simulink library "IAM_b0"  (Simulink 8.2)
settings: Solver=ode45  StartTime=0.0  StopTime=10.0  RelTol=1e-3
libraries: simulink x1, simulink_extras x1
settings Model: Creator=lena.frank  LastModifiedBy=drhf

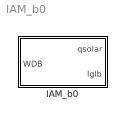
== system IAM_b0 ==
  IAM_b0 : Subsystem  mask(collector optics single glazing with extra white glass){fta=0.8, b0=0.12, Kd=0.92}
      mask prompts: fta "Fin Efficiency * Transmission * Absorption (FTA) [-]"; b0 "b0 : constant for the calculation of the incident angle modifier (direct radiation) [-]"; Kd "Kd : Incidence angle modifier diffuse radiation [-]"
      mask help:
      | USE IN THE "Collector_EN12975_FlatPlate" MODEL:
      | Transforms direct and diffuse radiation to an absorbed solar power per unit area. The direct radiation incidence angle modifier (Kdir) uses the b0-model for flat plate collectors (EN 12975).
      | FTA or F'(TauAlfa) is defined from the incidence angle modifiers Kdir and Kdfu:
      | FTA = eta0 / (Kdir(15°)*0.85 + Kdfu*0.15)
      mask Help: web(fullfile(path_carnot('help'),'IAM_b0.html'),'-helpbrowser')

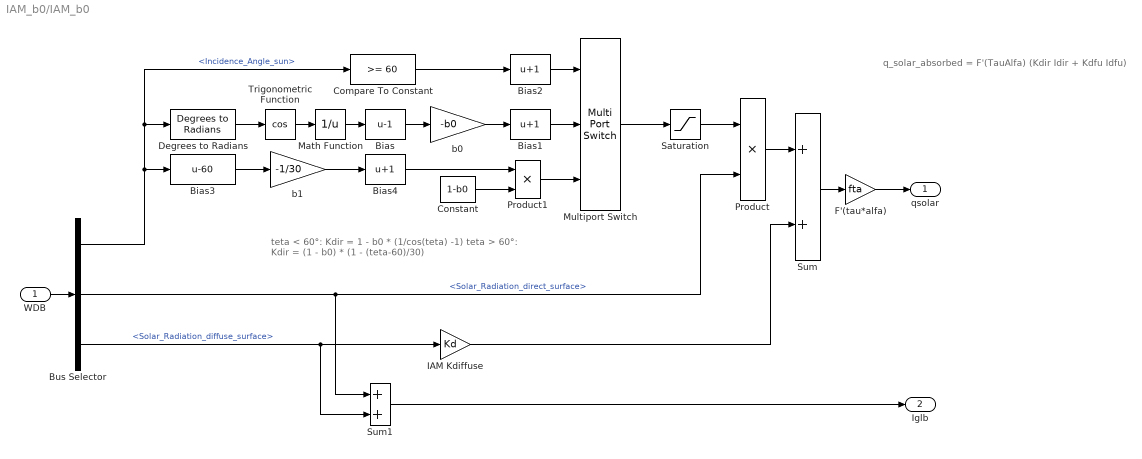
== system IAM_b0/IAM_b0 ==
  note: q_solar_absorbed = F'(TauAlfa) (Kdir Idir + Kdfu Idfu)
  note: teta < 60°: Kdir = 1 - b0 * (1/cos(teta) -1)
      | teta > 60°: Kdir = (1 - b0) * (1 - (teta-60)/30)
  WDB : Inport
  Bias : Bias  Bias=-1
  Bias1 : Bias  Bias=1
  Bias2 : Bias  Bias=1
  Bias3 : Bias  Bias=-60
  Bias4 : Bias  Bias=1
  Bus Selector : BusSelector  OutputSignals=Incidence_Angle_sun,Solar_Radiation_direct_surface,Solar_Radiation_diffuse_surface
  Compare To Constant : simulink/Logic and Bit Operations/Compare To Constant  relop=>=  const=60  OutDataTypeStr=uint8
  Constant : Constant  Value=1-b0
  Degrees to Radians : simulink_extras/Transformations/Degrees to Radians
  F'(tau*alfa) : Gain  Gain=fta  SaturateOnIntegerOverflow=on  OutDataTypeStr=Inherit: Same as input  ParamDataTypeStr=Inherit: Same as input
  IAM Kdiffuse : Gain  Gain=Kd  SaturateOnIntegerOverflow=on  OutDataTypeStr=Inherit: Same as input  ParamDataTypeStr=Inherit: Same as input
  Math Function : Math  Operator=reciprocal  SaturateOnIntegerOverflow=on
  Multiport Switch : MultiPortSwitch  Inputs=2
  Product : Product  RndMeth=Zero
  Product1 : Product  RndMeth=Zero
  Saturation : Saturate  UpperLimit=inf  LowerLimit=0
  Sum : Sum  SaturateOnIntegerOverflow=on  InputSameDT=on  OutDataTypeStr=Inherit: Same as first input
  Sum1 : Sum  SaturateOnIntegerOverflow=on  InputSameDT=on  OutDataTypeStr=Inherit: Same as first input
  Trigonometric Function : Trigonometry  Operator=cos
  b0 : Gain  Gain=-b0  SaturateOnIntegerOverflow=on  OutDataTypeStr=Inherit: Same as input  ParamDataTypeStr=Inherit: Same as input
  b1 : Gain  Gain=-1/30  SaturateOnIntegerOverflow=on  OutDataTypeStr=Inherit: Same as input  ParamDataTypeStr=Inherit: Same as input
  qsolar : Outport
  Iglb : Outport  Port=2
  wires:
  b0/1 -> Bias1/1
  Bias/1 -> b0/1
  Math Function/1 -> Bias/1
  Trigonometric Function/1 -> Math Function/1
  Degrees to Radians/1 -> Trigonometric Function/1
  Sum1/1 -> Iglb/1
  F'(tau*alfa)/1 -> qsolar/1
  Sum/1 -> F'(tau*alfa)/1
  Product/1 -> Sum/1
  IAM Kdiffuse/1 -> Sum/2
  Bus Selector/2 -> Sum1/1, Product/2  "<Solar_Radiation_direct_surface>"
  Bus Selector/1 -> Bias3/1, Compare To Constant/1, Degrees to Radians/1  "<Incidence_Angle_sun>"
  Bus Selector/3 -> Sum1/2, IAM Kdiffuse/1  "<Solar_Radiation_diffuse_surface>"
  WDB/1 -> Bus Selector/1
  Saturation/1 -> Product/1
  Compare To Constant/1 -> Bias2/1
  Bias2/1 -> Multiport Switch/1
  Bias1/1 -> Multiport Switch/2
  Multiport Switch/1 -> Saturation/1
  Bias3/1 -> b1/1
  b1/1 -> Bias4/1
  Constant/1 -> Product1/2
  Product1/1 -> Multiport Switch/3
  Bias4/1 -> Product1/1
